simulink model "compass"  (R2018a)
settings: Solver=VariableStepAuto  StartTime=0.0  StopTime=10.0  RelTol=1e-3
libraries: simulink_extras x1
settings Model: Creator=David  LastModifiedBy=David

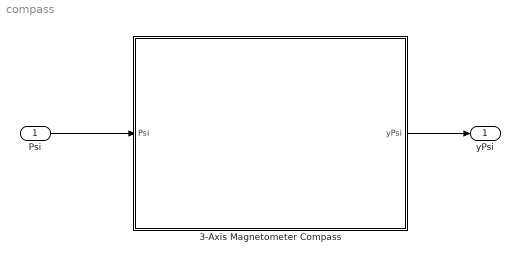
== system compass ==
  Psi : Inport
  3-Axis Magnetometer Compass : Subsystem  mask{SampleTime=1, headingNoiseDensity=0, headingBandwidthHz=1E06, headingInit=0, headingUpperSaturation=inf, headingLowerSaturation=-inf, headingResolution=1E-06}
      mask prompts: SampleTime "Magnetometer Sample Time (s)"; headingNoiseDensity "Magnetometer Heading Noise Density (rad/sqrt(Hz))"; headingBandwidthHz "Magnetometer Heading Sensor Bandwidth (Hz)"; headingInit "Magnetometer Heading Sensor Initial Condition (rad)"; headingUpperSaturation "Magnetometer Heading Sensor Upper Saturation Limit (rad)"; headingLowerSaturation "Magnetometer Heading Sensor Lower Saturation Limit (rad)"; headingResolution "Magnetometer Heading Sensor Resolution (rad)"
      mask DialogControl DescGroupVar Prompt: MEMS Magnetometer Model
      mask DialogControl DescTextVar Prompt: MEMS Magnetometer Model to Estimate Heading Angle with White Noise Modelling
      mask DialogControl Container7 Prompt: System Characteristics
      mask DialogControl Container4 Prompt: Noise Characteristics
      mask DialogControl Container6 Prompt: Sensor Dynamics
      mask DialogControl Container10 Prompt: Bandwidth
      mask DialogControl Container11 Prompt: Initial Conditions
      mask DialogControl Container8 Prompt: Limits and Quantization
      mask DialogControl Container13 Prompt: Limits
      mask DialogControl Container14 Prompt: Quantization
      mask Display:
      | image('mems_compass.jpg')
      | 
      | color('red')
      | 
      | port_label('input', 1, '\psi (rad)', 'texMode', 'on')
      | 
      | port_label('output', 1, 'y_{\psi} (rad)', 'texMode', 'on')
  yPsi : Outport
  wires:
  3-Axis Magnetometer Compass/1(yPsi) -> yPsi/1
  Psi/1 -> 3-Axis Magnetometer Compass/1(Psi)

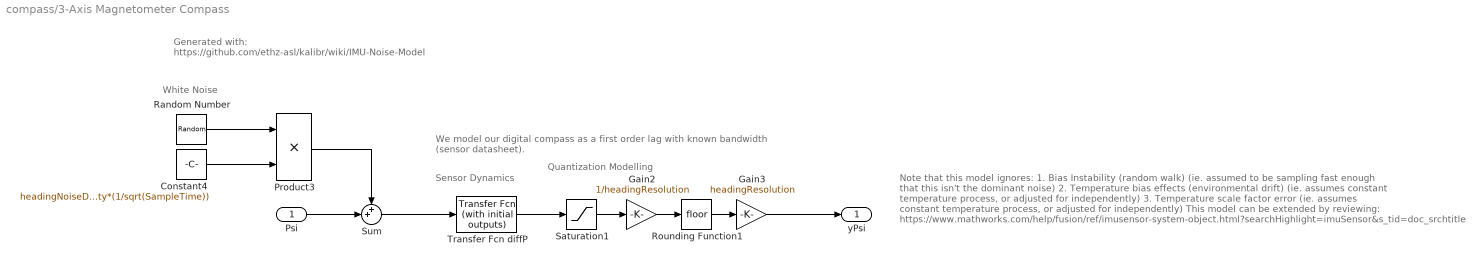
== system compass/3-Axis Magnetometer Compass ==
  note: White Noise
  note: Generated with:
      | https://github.com/ethz-asl/kalibr/wiki/IMU-Noise-Model
  note: Quantization Modelling
  note: We model our digital compass as a first order lag with known bandwidth
      | (sensor datasheet).
  note: Sensor Dynamics
  note: Note that this model ignores:
      | 1. Bias Instability (random walk) (ie. assumed to be sampling fast enough that this isn't the dominant noise)
      | 2. Temperature bias effects (environmental drift) (ie. assumes constant temperature process, or adjusted for independently)
      | 3. Temperature scale factor error (ie. assumes constant temperature process, or adjusted for independently)
      |
      | This model can be extended by reviewing:
      | https://www.mathworks.com/help/fusion/ref/imusensor-system-object.html?searchHighlight=imuSensor&s_tid=doc_srchtitle
  Psi : Inport
  Constant4 : Constant  Value=headingNoiseDensity*(1/sqrt(SampleTime))
  Gain2 : Gain  Gain=1/headingResolution
  Gain3 : Gain  Gain=headingResolution
  Product3 : Product
  Random Number : RandomNumber  SampleTime=SampleTime
  Rounding Function1 : Rounding
  Saturation1 : Saturate  UpperLimit=headingUpperSaturation  LowerLimit=headingLowerSaturation
  Sum : Sum  Inputs=++|
  Transfer Fcn diffP : simulink_extras/Additional Linear/Transfer Fcn (with initial outputs)  N=[headingBandwidthHz*2*pi]  D="[1,  headingBandwidthHz*2*pi]"  Y0=headingInit  U0=headingInit
  yPsi : Outport
  wires:
  Psi/1 -> Sum/2
  Random Number/1 -> Product3/1
  Product3/1 -> Sum/1
  Constant4/1 -> Product3/2
  Sum/1 -> Transfer Fcn diffP/1
  Rounding Function1/1 -> Gain3/1
  Gain2/1 -> Rounding Function1/1
  Saturation1/1 -> Gain2/1
  Transfer Fcn diffP/1 -> Saturation1/1
  Gain3/1 -> yPsi/1
